simulink model "model_ciagly"  (R2019b)
settings: Solver=VariableStepAuto  StartTime=0.0  StopTime=10.0  RelTol=1e-3
values from neighbouring files (symbols this model uses):
  Imax = lambda*In    [dane.m]
  J = 6    [dane.m]
  Kp = 0.15*Un    (= 33)    [dane.m]    (also in regulatory.m = kz)
  Kt = 10/(1.2*omega_n)    (= 0.0530516476973)    [dane.m]
  psi_en = (Un-Rt*In)/omega_n    (= 1.31652968926)    [dane.m]
  Rt = 0.15    [dane.m]
  T = Lt/Rt    [model_silnika.m]    (also in regulatory.m; regulatory_ciagle.m)
  Un = 220    [dane.m]
  Y = 10/(2.5*In)    (= 0.0454545454545)    [dane.m]
undefined symbols (not defined in the file or in its folder): Kw, m, u_z0, V
settings Model: Creator=jakub  LastModifiedBy=jakub
settings DataIOCC: SaveFormat=Array

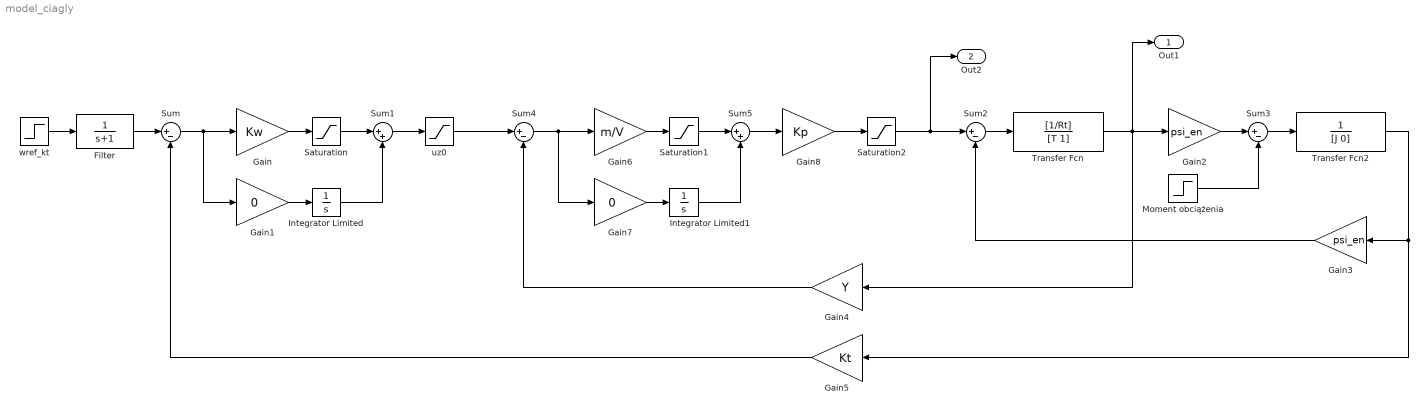
== system model_ciagly ==
  "Filter " : TransferFcn  Denominator=[1 1]
  Gain : Gain  Gain=Kw
  Gain1 : Gain  Gain=0
  Gain2 : Gain  Gain=psi_en
  Gain3 : Gain  Gain=psi_en
  Gain4 : Gain  Gain=Y
  Gain5 : Gain  Gain=Kt
  Gain6 : Gain  Gain=m/V
  Gain7 : Gain  Gain=0
  Gain8 : Gain  Gain=Kp
  Integrator Limited : Integrator  LimitOutput=on  UpperSaturationLimit=1  LowerSaturationLimit=0
  Integrator Limited1 : Integrator  LimitOutput=on  UpperSaturationLimit=1  LowerSaturationLimit=0
  Moment obciążenia : Step  SampleTime=0
  Saturation : Saturate  UpperLimit=u_z0  LowerLimit=-u_z0
  Saturation1 : Saturate  UpperLimit=Imax  LowerLimit=-Imax
  Saturation2 : Saturate  UpperLimit=Un  LowerLimit=-Un
  Sum{,2..4} (4 alike) : Sum  Inputs=|+-
  Sum1 : Sum  Inputs=|++
  Sum5 : Sum  Inputs=|++
  Transfer Fcn : TransferFcn  Numerator=[1/Rt]  Denominator=[T 1]
  Transfer Fcn2 : TransferFcn  Denominator=[J 0]
  uz0 : Saturate  UpperLimit=u_z0  LowerLimit=-u_z0
  wref_kt : Step  SampleTime=0
  Out1 : Outport
  Out2 : Outport  Port=2
  wires:
  wref_kt/1 -> "Filter "/1
  "Filter "/1 -> Sum/1
  Sum/1 -> Gain1/1, Gain/1
  Gain/1 -> Saturation/1
  Gain1/1 -> Integrator Limited/1
  Saturation/1 -> Sum1/1
  Integrator Limited/1 -> Sum1/2
  Sum1/1 -> uz0/1
  Sum2/1 -> Transfer Fcn/1
  Transfer Fcn/1 -> Gain4/1, Out1/1, Gain2/1
  Gain2/1 -> Sum3/1
  Moment obciążenia/1 -> Sum3/2
  Sum3/1 -> Transfer Fcn2/1
  Gain3/1 -> Sum2/2
  Transfer Fcn2/1 -> Gain3/1, Gain5/1
  Sum4/1 -> Gain7/1, Gain6/1
  Gain6/1 -> Saturation1/1
  uz0/1 -> Sum4/1
  Gain7/1 -> Integrator Limited1/1
  Saturation1/1 -> Sum5/1
  Integrator Limited1/1 -> Sum5/2
  Sum5/1 -> Gain8/1
  Gain8/1 -> Saturation2/1
  Saturation2/1 -> Out2/1, Sum2/1
  Gain4/1 -> Sum4/2
  Gain5/1 -> Sum/2
